simulink model "Camara_de_frio"  (R2021a)
settings: Solver=VariableStepAuto  StartTime=0.0  StopTime=2000000  RelTol=1e-3
settings Model: Creator=Manu  LastModifiedBy=franc

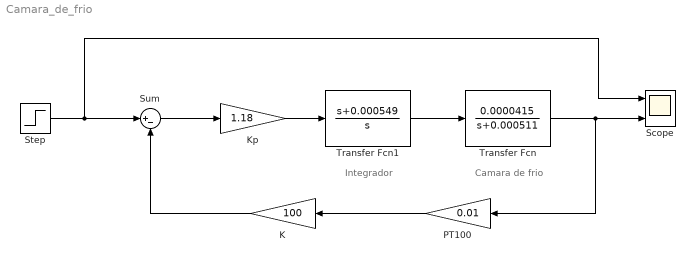
== system Camara_de_frio ==
  note: Integrador
  note: Camara de frio
  K : Gain  Gain=100
  Kp : Gain  Gain=1.18
  PT100 : Gain  Gain=0.01
  Scope : Scope  NumInputPorts=2
  Step : Step  Time=1000000  Before=25  After=-5  SampleTime=0
  Sum : Sum  Inputs=|+-
  Transfer Fcn : TransferFcn  Numerator=[0.0000415]  Denominator=[1 0.000511]
  Transfer Fcn1 : TransferFcn  Numerator=[1 0.000549]  Denominator=[1 0]
  wires:
  Transfer Fcn1/1 -> Transfer Fcn/1
  K/1 -> Sum/2
  Transfer Fcn/1 -> PT100/1, Scope/2
  Step/1 -> Sum/1, Scope/1
  Kp/1 -> Transfer Fcn1/1
  Sum/1 -> Kp/1
  PT100/1 -> K/1
